simulink model "verify_Pump_Simple_mdl"  (R2016b)
settings: Solver=ode45  StartTime=0.0  StopTime=75  MaxStep=1  RelTol=1e-3  EnableMultiTasking=on
libraries: carnot x2, simulink x1
settings Model: Creator=drhf  LastModifiedBy=drhf
settings DataIOCC: SaveFormat=Array  SignalLoggingSaveFormat=ModelDataLogs
settings OptimizationCC: ExpressionDepthLimit=2147483647  LifeSpan=inf
settings DebuggingCC: UnderspecifiedInitializationDetection=Classic  MergeDetectMultiDrivingBlocksExec=none  SolverPrmCheckMsg=warning  FcnCallInpInsideContextMsg=warning  StateNameClashWarn=warning  SFUnexpectedBacktrackingDiag=warning  SFNoUnconditionalDefaultTransitionDiag=warning  SFExecutionAtInitializationDiag=none
settings HardwareCC: ProdBitPerPointer=32  ProdBitPerSizeT=32  ProdBitPerPtrDiffT=32  ProdLargestAtomicFloat=None  ProdIntDivRoundTo=Undefined  ProdEndianess=Unspecified  ProdWordSize=32  ProdHWDeviceType=32-bit Generic
settings ModelReferenceCC: PropagateSignalLabelsOutOfModel=off
settings GRTTargetCC: TargetLangStandard=C89/C90 (ANSI)  GeneratePreprocessorConditionals=Disable all  CombineOutputUpdateFcns=off  GRTInterface=on
settings ConfigComp: CovMetricSettings=dw  CovHtmlReporting=on  CovSaveCumulativeToWorkspaceVar=on  CovSaveSingleToWorkspaceVar=on  CovExternalEMLEnable=off

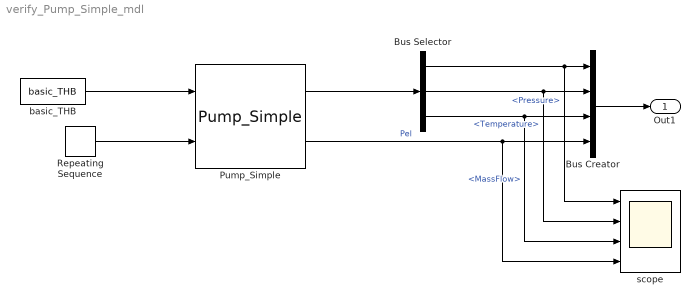
== system verify_Pump_Simple_mdl ==
  Bus Creator : BusCreator  Inputs=4
  Bus Selector : BusSelector  OutputSignals=Pressure,Temperature,MassFlow
  Pump_Simple : carnot/Hydraulics/Pump_Simple  mdotmax=1200/3600  dia=0.0157  power=30  fluid_id=Water  mix=0  p0=3e5
  Repeating Sequence : simulink/Sources/Repeating Sequence  rep_seq_t=[0 20 60 80]  rep_seq_y=[0 0 1 1]
  basic_THB : carnot/Basic/Hydraulics/basic_THB  t=20  mdot=700/3600  p=1e5  ID=Pressure Drop from Massflow  fluid=Water  mix=0  mix2=0  mix3=0  dia=0.02  hgt=0
  scope : Scope  NumInputPorts=4
  Out1 : Outport
  wires:
  Bus Creator/1 -> Out1/1
  Bus Selector/3 -> scope/3, Bus Creator/3  "<MassFlow>"
  Repeating Sequence/1 -> Pump_Simple/2
  Pump_Simple/1 -> Bus Selector/1
  Pump_Simple/2 -> scope/4, Bus Creator/4  "Pel"
  Bus Selector/1 -> scope/1, Bus Creator/1  "<Pressure>"
  Bus Selector/2 -> scope/2, Bus Creator/2  "<Temperature>"
  basic_THB/1 -> Pump_Simple/1
